simulink model "EX5_zadanie2"  (R2023b)
settings: Solver=FixedStepDiscrete  StartTime=0.0  StopTime=0  RelTol=1e-3
libraries: CPOiS_SourcesSinks x6, CPOiS_LinearTransforms x4, CPOiS_DataManipulation_DataTypeConversion x2, CPOiS_Edges x1
settings Model: Creator=alyskawa  LastModifiedBy=alyskawa

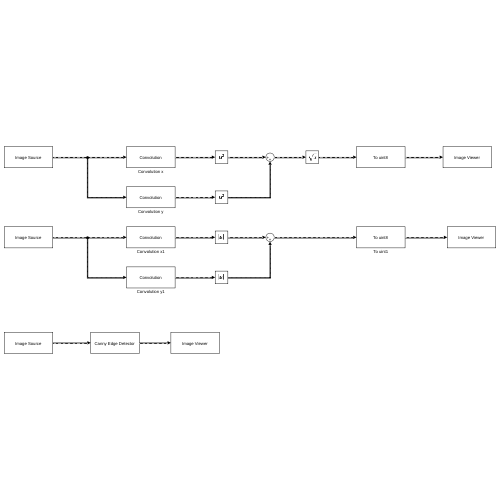
[thumbnail: Simulink's stored preview of the top-level diagram]
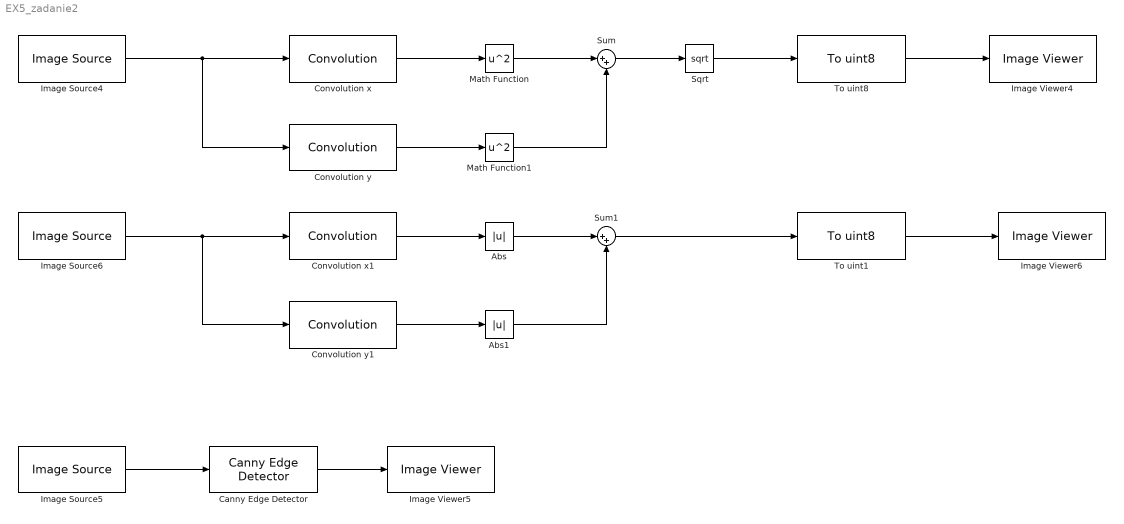
== system EX5_zadanie2 ==
  Abs : Abs  SaturateOnIntegerOverflow=off
  Abs1 : Abs  SaturateOnIntegerOverflow=off
  Canny Edge Detector : CPOiS_Edges/Canny Edge Detector  LowThresh=0  HighThresh=30
      settings: SourceProductName=CPOiS - Digital image and signal processing
  Convolution x : CPOiS_LinearTransforms/Convolution  ConvolutionMatrix=[-1,0,1;-2,0,2;-1,0,1]
      settings: SourceProductName=CPOiS - Digital image and signal processing
  Convolution x1 : CPOiS_LinearTransforms/Convolution  ConvolutionMatrix=[-1,0,1;-2,0,2;-1,0,1]
      settings: SourceProductName=CPOiS - Digital image and signal processing
  Convolution y : CPOiS_LinearTransforms/Convolution  ConvolutionMatrix=[-1,-2,-1;0,0,0;1,2,1]
      settings: SourceProductName=CPOiS - Digital image and signal processing
  Convolution y1 : CPOiS_LinearTransforms/Convolution  ConvolutionMatrix=[-1,-2,-1;0,0,0;1,2,1]
      settings: SourceProductName=CPOiS - Digital image and signal processing
  Image Source4 : CPOiS_SourcesSinks/Image Source  FileSelection=ball.png
      settings: SourceProductName=CPOiS - Digital image and signal processing
  Image Source5 : CPOiS_SourcesSinks/Image Source  FileSelection=ball.png
      settings: SourceProductName=CPOiS - Digital image and signal processing
  Image Source6 : CPOiS_SourcesSinks/Image Source  FileSelection=ball.png
      settings: SourceProductName=CPOiS - Digital image and signal processing
  Image Viewer4 : CPOiS_SourcesSinks/Image Viewer
      settings: SourceProductName=CPOiS - Digital image and signal processing
  Image Viewer5 : CPOiS_SourcesSinks/Image Viewer
      settings: SourceProductName=CPOiS - Digital image and signal processing
  Image Viewer6 : CPOiS_SourcesSinks/Image Viewer
      settings: SourceProductName=CPOiS - Digital image and signal processing
  Math Function : Math  Operator=square
  Math Function1 : Math  Operator=square
  Sqrt : Sqrt
  Sum : Sum  Inputs=|++
  Sum1 : Sum  Inputs=|++
  To uint1 : CPOiS_DataManipulation_DataTypeConversion/To uint8
      settings: SourceProductName=CPOiS - Digital image and signal processing
  To uint8 : CPOiS_DataManipulation_DataTypeConversion/To uint8
      settings: SourceProductName=CPOiS - Digital image and signal processing
  wires:
  To uint8/1 -> Image Viewer4/1
  Convolution y1/1 -> Abs1/1
  Abs1/1 -> Sum1/2
  To uint1/1 -> Image Viewer6/1
  Convolution y/1 -> Math Function1/1
  Sqrt/1 -> To uint8/1
  Abs/1 -> Sum1/1
  Convolution x/1 -> Math Function/1
  Math Function/1 -> Sum/1
  Image Source4/1 -> Convolution y/1, Convolution x/1
  Sum/1 -> Sqrt/1
  Math Function1/1 -> Sum/2
  Image Source6/1 -> Convolution y1/1, Convolution x1/1
  Convolution x1/1 -> Abs/1
  Sum1/1 -> To uint1/1
  Canny Edge Detector/1 -> Image Viewer5/1
  Image Source5/1 -> Canny Edge Detector/1
